simulink subsystem "HIL_Send_TCP_Data_2021a1"  (R2021a)
settings: Solver=VariableStepAuto  StartTime=0.0  StopTime=10.0  RelTol=1e-3
model mask{mi_ip=mi_ip, mi_port=mi_port, f=0}
  mask prompts: mi_ip "Server IP"; mi_port "Server Port"; f "Sampling Frequency"
libraries: slrealtimeiplib x2
settings Model: Creator=ramuj  LastModifiedBy=ramuj
settings DebuggingCC: UnconnectedInputMsg=none  UnconnectedOutputMsg=none  UnconnectedLineMsg=none
settings ModelReferenceCC: EnableRefExpFcnMdlSchedulingChecks=off
settings RTWCC: Description=Generic Real-Time Target  DLArmComputeVersion=20.02.1

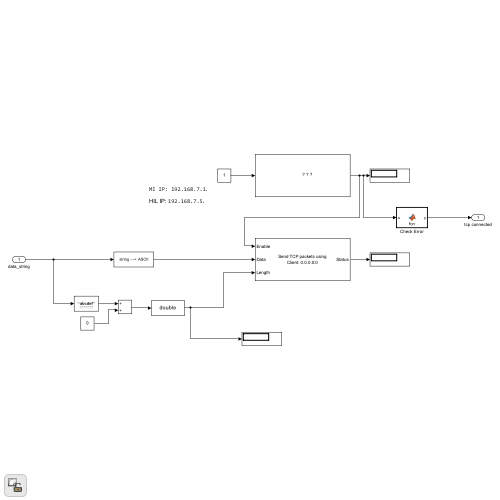
[thumbnail: Simulink's stored preview of the top-level diagram]
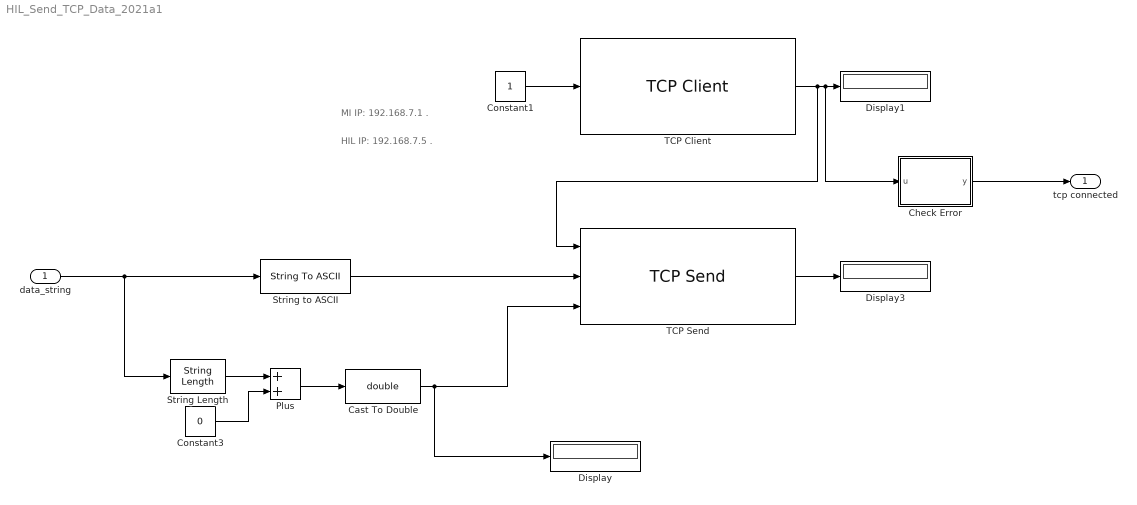
== system HIL_Send_TCP_Data_2021a1 ==
  note: MI IP: 192.168.7.1 .
  note: HIL IP: 192.168.7.5 .
  data_string : Inport
  Cast To Double : DataTypeConversion  OutDataTypeStr=double
  Check Error : MATLAB Function  TreatAsAtomicUnit=on
  Constant1 : Constant
  Constant3 : Constant  Value=0
  Display : Display
  Display1 : Display
  Display3 : Display
  Plus : Sum
  String Length : StringLength
  String to ASCII : StringToASCII
  TCP Client : slrealtimeiplib/TCP Client  Priority=-1  useHostTargetConn=off  remoteAddress=mi_ip  remotePort=mi_port  clientAddress=0.0.0.0  clientPort=0
  TCP Send : slrealtimeiplib/TCP Send  socketAddPortVal=Client: 0.0.0.0:0  sampleTime=1/f
  tcp connected : Outport
  wires:
  String Length/1 -> Plus/1
  Cast To Double/1 -> TCP Send/3, Display/1
  Plus/1 -> Cast To Double/1
  Check Error/1(y) -> tcp connected/1
  data_string/1 -> String Length/1, String to ASCII/1
  Constant1/1 -> TCP Client/1
  TCP Client/1 -> TCP Send/1, Check Error/1(u), Display1/1
  TCP Send/1 -> Display3/1
  String to ASCII/1 -> TCP Send/2
  Constant3/1 -> Plus/2

== matlab function HIL_Send_TCP_Data_2021a1/Check Error ==
  data: u input; y output
function y = fcn(u)

    if(u == 1)
        y = "Connected";
    else 
        y = "Error";
    end
end
